simulink model "SimPunto1"  (R2024b)
settings: Solver=VariableStepAuto  StartTime=0.0  StopTime=30  RelTol=1e-3
values from neighbouring files (symbols this model uses):
  den = [1 0.594985 321.255843 0]    [c2d.m]
  num = [0.370465 0.265128 118.983645]    [c2d.m]
undefined symbols (not defined in the file or in its folder): dend, denr, dspblkCoreblockFVToolHelper, gcbh, numd, numr

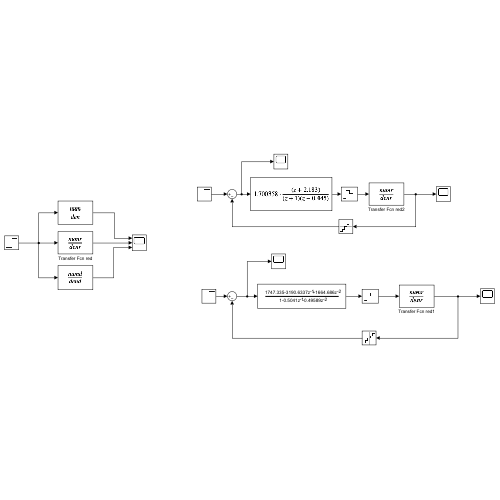
[thumbnail: Simulink's stored preview of the top-level diagram]
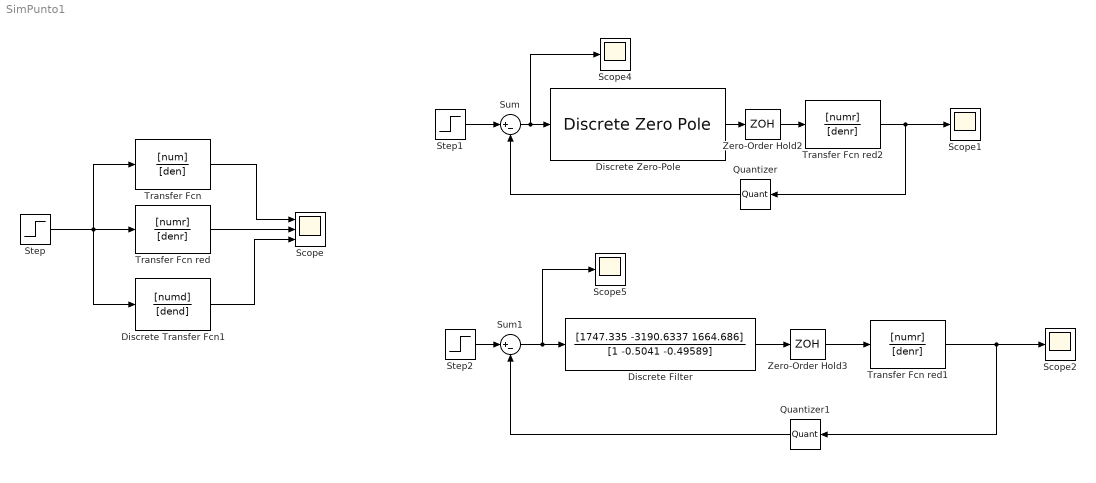
== system SimPunto1 ==
  Discrete Transfer Fcn1 : DiscreteTransferFcn  LoadFcn=dspblkCoreblockFVToolHelper(gcbh,'load');  Numerator=[numd]  Denominator=[dend]
  Discrete Zero-Pole : DiscreteZeroPole  Zeros=[-2.183]  Poles=[-1 0.445]  Gain=1.700358  SampleTime=-1
  Discrete Filter : DiscreteFilter  LoadFcn=dspblkCoreblockFVToolHelper(gcbh,'load');  Numerator=[1747.335 -3190.6337 1664.686]  Denominator=[1 -0.5041 -0.49589]
  Quantizer : Quantizer  QuantizationInterval=3.3/1024
  Quantizer1 : Quantizer  QuantizationInterval=3.3/1024
  Scope : Scope  NumInputPorts=3
  Scope{1..2,4..5} (4 alike) : Scope
  Step : Step  Time=0  SampleTime=0
  Step1 : Step  SampleTime=0
  Step2 : Step  Time=0  SampleTime=0
  Sum : Sum  Inputs=|+-
  Sum1 : Sum  Inputs=|+-
  Transfer Fcn : TransferFcn  Numerator=[num]  Denominator=[den]
  Transfer Fcn red : TransferFcn  Numerator=[numr]  Denominator=[denr]
  Transfer Fcn red1 : TransferFcn  Numerator=[numr]  Denominator=[denr]
  Transfer Fcn red2 : TransferFcn  Numerator=[numr]  Denominator=[denr]
  Zero-Order Hold2 : ZeroOrderHold  SampleTime=0.1
  Zero-Order Hold3 : ZeroOrderHold  SampleTime=0.1
  wires:
  Transfer Fcn red1/1 -> Scope2/1, Quantizer1/1
  Sum/1 -> Discrete Zero-Pole/1, Scope4/1
  Quantizer/1 -> Sum/2
  Step2/1 -> Sum1/1
  Step1/1 -> Sum/1
  Transfer Fcn red2/1 -> Scope1/1, Quantizer/1
  Discrete Zero-Pole/1 -> Zero-Order Hold2/1
  Zero-Order Hold2/1 -> Transfer Fcn red2/1
  Transfer Fcn red/1 -> Scope/2
  Discrete Transfer Fcn1/1 -> Scope/3
  Step/1 -> Transfer Fcn/1, Discrete Transfer Fcn1/1, Transfer Fcn red/1
  Transfer Fcn/1 -> Scope/1
  Quantizer1/1 -> Sum1/2
  Zero-Order Hold3/1 -> Transfer Fcn red1/1
  Discrete Filter/1 -> Zero-Order Hold3/1
  Sum1/1 -> Scope5/1, Discrete Filter/1
